simulink model "pid_controller_test"  (R2024b)
settings: Solver=ode1  StartTime=0.0  StopTime=20  FixedStep=dt  RelTol=1e-3
model workspace (MAT data in the model file):
  Kd = 5
  Ki = 20
  Kp = 20
  N = 0
  Sig = Simulink.Signal
  Sig.Dimensions = -1
  Sig.DimensionsMode = 'auto'
  Sig.Complexity = 'auto'
  Sig.SampleTime = -1
  Sig.SamplingMode = 'auto'
  Sig.DataType = 'auto'
  dt = 0.0001
libraries: slpidlib x1
settings Model: Creator=emil  LastModifiedBy=emil
settings RTWCC: GPUComputeCapability=3.5

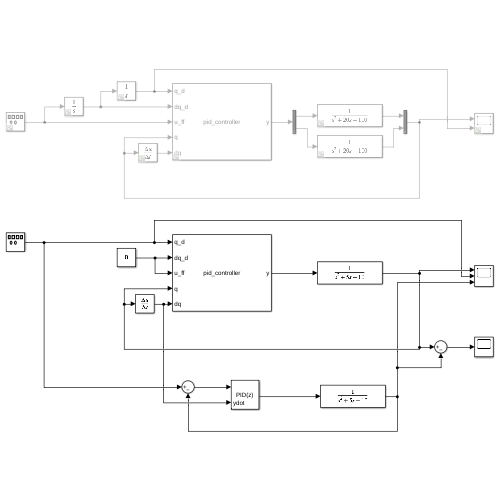
[thumbnail: Simulink's stored preview of the top-level diagram]
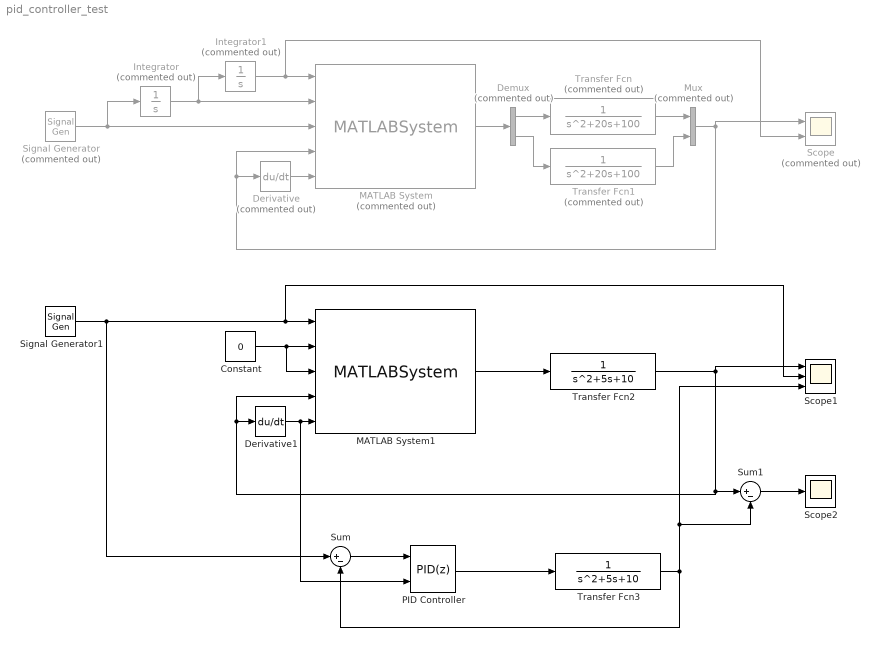
== system pid_controller_test ==
  Constant : Constant  Value=0
  Demux : Demux  Commented=on  Outputs=2
  Derivative : Derivative  Commented=on
  Derivative1 : Derivative
  Integrator : Integrator  Commented=on
  Integrator1 : Integrator  Commented=on
  MATLAB System : MATLABSystem  Commented=on  System=pid_controller  Kp=Kp  Ki=Ki  Kd=Kd  N=1  num_states=2  sample_time=dt  SimulateUsing=Interpreted execution
      mask Type: pid_controller
      mask Display:
      | disp('pid_controller');
      | port_label('input',1,'q_d');
      | port_label('input',2,'dq_d');
      | port_label('input',3,'u_ff');
      | port_label('input',4,'q');
      | port_label('input',5,'dq');
      | port_label('output',1,'y');
  MATLAB System1 : MATLABSystem  System=pid_controller  Kp=Kp  Ki=Ki  Kd=Kd  N=1  num_states=1  sample_time=dt  SimulateUsing=Interpreted execution
      mask Type: pid_controller
      mask Display:
      | disp('pid_controller');
      | port_label('input',1,'q_d');
      | port_label('input',2,'dq_d');
      | port_label('input',3,'u_ff');
      | port_label('input',4,'q');
      | port_label('input',5,'dq');
      | port_label('output',1,'y');
  Mux : Mux  Commented=on  Inputs=2
  PID Controller : slpidlib/PID Controller  Controller=PID  Form=Parallel  TimeDomain=Discrete-time  UseExternalTs=off  SampleTime=dt  IntegratorMethod=Forward Euler  FilterMethod=Forward Euler  ControllerParametersSource=internal  P=Kp  I=Ki  UseKiTs=off  D=Kd  UseExternalDerivativeSource=on  N=100  UseFilter=off  TunerSelectOption=Transfer Function Based (PID Tuner App)  InitialConditionSource=internal  InitialConditionForIntegrator=0  InitialConditionForFilter=0  DifferentiatorICPrevScaledInput=0  ExternalReset=none  TrackingMode=off  Kt=1  LimitOutput=off  SatLimitsSource=internal  UpperSaturationLimit=inf  LowerSaturationLimit=-inf  LinearizeAsGain=on  AntiWindupMode=none  Kb=1  LimitIntegrator=off  UpperIntegratorSaturationLimit=inf  LowerIntegratorSaturationLimit=-inf  POutMin=[]  POutMax=[]  IOutMin=[]  IOutMax=[]  DOutMin=[]  DOutMax=[]  NOutMin=[]  NOutMax=[]  SumOutMin=[]  SumOutMax=[]  SaturationOutMin=[]  SaturationOutMax=[]  PParamMin=[]  PParamMax=[]  IParamMin=[]  IParamMax=[]  DParamMin=[]  DParamMax=[]  NParamMin=[]  NParamMax=[]  KbParamMin=[]  KbParamMax=[]  KtParamMin=[]  KtParamMax=[]  KbOutMin=[]  KbOutMax=[]  KtOutMin=[]  KtOutMax=[]  IntegratorOutMin=[]  IntegratorOutMax=[]  FilterOutMin=[]  FilterOutMax=[]  SumI1OutMin=[]  SumI1OutMax=[]  SumI2OutMin=[]  SumI2OutMax=[]  SumI3OutMin=[]  SumI3OutMax=[]  SumI4OutMin=[]  SumI4OutMax=[]  SumDOutMin=[]  SumDOutMax=[]  DifferentiatorOutMin=[]  DifferentiatorOutMax=[]  FilterDiffOutCoefMin=[]  FilterDiffOutCoefMax=[]  ReciprocalOutMin=[]  ReciprocalOutMax=[]  SumDenOutMin=[]  SumDenOutMax=[]  SumNumOutMin=[]  SumNumOutMax=[]  DivideOutMin=[]  DivideOutMax=[]  UdiffTsProdOutMin=[]  UdiffTsProdOutMax=[]  NTsProdOutMin=[]  NTsProdOutMax=[]  UintegralTsProdOutMin=[]  UintegralTsProdOutMax=[]  UngainTsProdOutMin=[]  UngainTsProdOutMax=[]  ClampingZeroOutDataTypeStr=Inherit: Inherit via back propagation  ClampingZeroOutMin=[]  ClampingZeroOutMax=[]  FilterDenConstantOutDataTypeStr=Inherit: Inherit via back propagation  FilterDenConstantOutMin=[]  FilterDenConstantOutMax=[]  PCopyOutDataTypeStr=Inherit: Inherit via back propagation  PCopyOutMin=[]  PCopyOutMax=[]  NCopyOutDataTypeStr=Inherit: Inherit via back propagation  NCopyOutMin=[]  NCopyOutMax=[]  IntegratorContinuousStateAttributes=''  IntegratorStateMustResolveToSignalObject=off  IntegratorRTWStateStorageClass=Auto  FilterContinuousStateAttributes=''  FilterStateMustResolveToSignalObject=off  FilterRTWStateStorageClass=Auto  ParallelPVariant=InternalParameters  IdealPVariant=Disabled  IVariant=InternalParameters  DVariant=InternalParameters  IntegratorVariant=Discrete  SatVariant=Disabled  AWVariant=Passthrough  PCopyVariant=Disabled  TRVariant=Disabled  FdbkBlocksVariant=Forward  IdealPFdbkVariant=Disabled  SatFdbkVariant=Disabled  DerivativeFilterVariant=Passthrough  NVariant=Passthrough  NCopyVariant=Disabled_SignalSpec  FilterICVariant=Disabled  IntegratorICVariant=InternalICs  ExternalResetVariant=Disabled  TRSumVariant=Passthrough  SumFdbkVariant=Disabled  SumVariant=Sum_PID  TsampFilterVariant=InternalTs  TsampNgainVariant=Passthrough  TsampIntegralVariant=Disabled_SignalSpec  ExternalSaturationOutDataTypeStr=Inherit: Same as second input  DerivativeSourceVariant=ExternalYdot  PreIntVariant=InternalPreInt
  Scope : Scope  Commented=on  NumInputPorts=2
  Scope1 : Scope  NumInputPorts=3
  Scope2 : Scope
  Signal Generator : SignalGenerator  Commented=on  Amplitude=[1 1] / 100  Frequency=[1 2] * 100  Units=rad/sec
  Signal Generator1 : SignalGenerator  WaveForm=square  Amplitude=0.1  Frequency=0.5  Units=rad/sec
  Sum : Sum  Inputs=|+-
  Sum1 : Sum  Inputs=|+-
  Transfer Fcn : TransferFcn  Commented=on  Denominator=[1 20 100]
  Transfer Fcn1 : TransferFcn  Commented=on  Denominator=[1 20 100]
  Transfer Fcn2 : TransferFcn  Denominator=[1 5 10]
  Transfer Fcn3 : TransferFcn  Denominator=[1 5 10]
  wires:
  Signal Generator/1 -> Integrator/1, MATLAB System/3
  Integrator1/1 -> Scope/2, MATLAB System/1
  Integrator/1 -> Integrator1/1, MATLAB System/2
  MATLAB System/1 -> Demux/1
  Derivative/1 -> MATLAB System/5
  Transfer Fcn/1 -> Mux/1
  Transfer Fcn1/1 -> Mux/2
  Mux/1 -> MATLAB System/4, Derivative/1, Scope/1
  Demux/1 -> Transfer Fcn/1
  Demux/2 -> Transfer Fcn1/1
  Transfer Fcn2/1 -> MATLAB System1/4, Derivative1/1, Sum1/1, Scope1/1
  Derivative1/1 -> PID Controller/2, MATLAB System1/5
  MATLAB System1/1 -> Transfer Fcn2/1
  Signal Generator1/1 -> Sum/1, Scope1/2, MATLAB System1/1
  Constant/1 -> MATLAB System1/3, MATLAB System1/2
  PID Controller/1 -> Transfer Fcn3/1
  Sum/1 -> PID Controller/1
  Transfer Fcn3/1 -> Sum/2, Sum1/2, Scope1/3
  Sum1/1 -> Scope2/1
